simulink model "Az5"  (R2020b)
settings: Solver=VariableStepAuto  StartTime=0.0  StopTime=10.0  RelTol=1e-3
settings Model: Creator=Mah  LastModifiedBy=admin

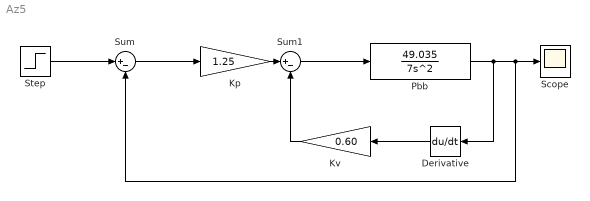
== system Az5 ==
  Derivative : Derivative
  Kp : Gain  Gain=1.25
  Kv : Gain  Gain=0.60
  Pbb : TransferFcn  Numerator=[49.035]  Denominator=[7 0 0]
  Scope : Scope
  Step : Step  SampleTime=0
  Sum : Sum  Inputs=|+-
  Sum1 : Sum  Inputs=|+-
  wires:
  Sum/1 -> Kp/1
  Step/1 -> Sum/1
  Kp/1 -> Sum1/1
  Derivative/1 -> Kv/1
  Pbb/1 -> Derivative/1, Sum/2, Scope/1
  Sum1/1 -> Pbb/1
  Kv/1 -> Sum1/2
